simulink model "Project"  (R2020a)
settings: Solver=FixedStepDiscrete  StartTime=0.0  StopTime=10.0  FixedStep=1.0  RelTol=1e-3
libraries: simulink x4
settings Model: Creator=Sajad  LastModifiedBy=alireza
settings OptimizationCC: DefaultParameterBehavior=Inlined  UseDivisionForNetSlopeComputation=on  GainParamInheritBuiltInType=on  UseFloatMulNetSlope=on  InlineInvariantSignals=on  PassReuseOutputArgsAs=Individual arguments  ZeroExternalMemoryAtStartup=off  ZeroInternalMemoryAtStartup=off  NoFixptDivByZeroProtection=on  EfficientFloat2IntCast=on  LifeSpan=1  OptimizeBlockOrder=speed  DifferentSizesBufferReuse=on  EfficientTunableParamExpr=on
settings DebuggingCC: ParameterTunabilityLossMsg=error
settings HardwareCC: ProdBitPerInt=16  ProdBitPerPointer=16  ProdBitPerSizeT=16  ProdBitPerPtrDiffT=16  ProdLargestAtomicFloat=None  ProdWordSize=8  ProdLongLongMode=on  ProdHWDeviceType=Atmel->AVR
settings SFSimCC: MATLABDynamicMemAlloc=off  CustomCodeUndefinedFunction=UseInterfaceOnly
settings RTWCC: SystemTargetFile=ert.tlc  GenCodeOnly=on  TemplateMakefile=ert_default_tmf  GenerateReport=on  IncludeHyperlinkInReport=on  LaunchReport=on  TargetLang=C++  GenerateTraceInfo=on  GenerateTraceReport=on  GenerateTraceReportSl=on  GenerateTraceReportSf=on  GenerateTraceReportEml=on
settings CodeAppCC: ForceParamTrailComments=on  IgnoreCustomStorageClasses=off  OperatorAnnotations=on  SimulinkDataObjDesc=on  SFDataObjDesc=on  CustomSymbolStrGlobalVar=rt$N$M  CustomSymbolStrType=$N$M  CustomSymbolStrFcn=$N$M$F  CustomSymbolStrMacro=$N$M  InsertBlockDesc=on
settings ERTTargetCC: TargetLangStandard=C++03 (ISO)  GenerateSampleERTMain=on  IncludeMdlTerminateFcn=off  CombineSignalStateStructs=on  SupportAbsoluteTime=off  MultiInstanceERTCode=on  CodeInterfacePackaging=C++ class  PurelyIntegerCode=on  SupportComplex=off  SupportNonInlinedSFcns=on  InlinedParameterPlacement=NonHierarchical  RootIOFormat=Structure reference  ERTCustomFileTemplate=example_file_process.tlc  ERTFilePackagingFormat=CompactWithDataFile

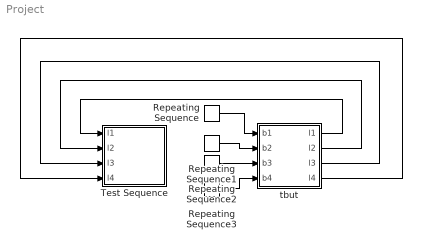
== system Project ==
  Repeating Sequence : simulink/Sources/Repeating Sequence  rep_seq_t=[0 1 2 3 4 5 6]  rep_seq_y=[0 1 1 0 0 0 0]
  Repeating Sequence1 : simulink/Sources/Repeating Sequence  rep_seq_t=[0 1 2 3 4 5 6]  rep_seq_y=[0 1 0 1 0 0 0]
  Repeating Sequence2 : simulink/Sources/Repeating Sequence  rep_seq_t=[0 1 2 3 4 5 6]  rep_seq_y=[0 1 0 0 1 0 0]
  Repeating Sequence3 : simulink/Sources/Repeating Sequence  rep_seq_t=[0 1 2 3 4 5 6]  rep_seq_y=[0 1 0 0 0 1 0]
  Test Sequence : Test Sequence  TreatAsAtomicUnit=on
  tbut : Stateflow chart  TreatAsAtomicUnit=on
  wires:
  tbut/1(l1) -> Test Sequence/1(l1)
  tbut/2(l2) -> Test Sequence/2(l2)
  tbut/3(l3) -> Test Sequence/3(l3)
  tbut/4(l4) -> Test Sequence/4(l4)
  Repeating Sequence/1 -> tbut/1(b1)
  Repeating Sequence3/1 -> tbut/4(b4)
  Repeating Sequence2/1 -> tbut/3(b3)
  Repeating Sequence1/1 -> tbut/2(b2)

== stateflow chart Project/tbut ==
  state fled_1 [parallel]
    settings: executionOrder=1
    state I
    state II
      l1 = ~l1;
    (default) -> fled_1.I
    fled_1.II -> fled_1.I [order 2]
    fled_1.I -> fled_1.II : [b1==1]
    fled_1.II -> fled_1.II [order 1] : [b1==1]
  state fled_2 [parallel]
    settings: executionOrder=2
    state I
    state II
      l2 = ~l2;
    (default) -> fled_2.I
    fled_2.II -> fled_2.I [order 2]
    fled_2.I -> fled_2.II : [b2==1]
    fled_2.II -> fled_2.II [order 1] : [b2==1]
  state fled_3 [parallel]
    settings: executionOrder=3
    state I
    state II
      l3 = ~l3;
    (default) -> fled_3.I
    fled_3.II -> fled_3.I [order 2]
    fled_3.I -> fled_3.II : [b3==1]
    fled_3.II -> fled_3.II [order 1] : [b3==1]
  state fled_4 [parallel]
    settings: executionOrder=4
    state I
    state II
      l4 = ~l4;
    (default) -> fled_4.I
    fled_4.II -> fled_4.I [order 2]
    fled_4.I -> fled_4.II : [b4==1]
    fled_4.II -> fled_4.II [order 1] : [b4==1]
  data: l1 output =false; l2 output =false; l3 output =false; l4 output =false; b1 input; b2 input; b3 input; b4 input

== stateflow chart Project/Test Sequence ==
  settings: stateMachineType=SIMPLIFIED_MACHINE
  state step_1
    verify(l1==false&& l2==false && l3==false && l4==false)
  state step_2
    verify(l1==true&& l2==true && l3==true && l4==true)
  state step_3
    verify(l1==false&& l2==true&& l3==true&& l4==true)
  state step_4
    verify(l1==false && l2==false && l3==true&& l4==true)
  state step_5
    verify(l1==false && l2==false&& l3==false&& l4==true)
  state step_6
    verify(l1==false&& l2==false && l3==false && l4==false)
  state step_7
  (default) -> step_1
  step_1 -> step_2 : [
      | after(1,sec)
      | ]
  step_2 -> step_3 : [
      | after(1,sec)
      | ]
  step_3 -> step_4 : [
      | after(1,sec)
      | ]
  step_4 -> step_5 : [
      | after(1,sec)
      | ]
  step_5 -> step_6 : [
      | after(1,sec)
      | ]
  step_6 -> step_7 : [
      | after(1,sec)
      | ]
  data: l1 input; l2 input; l3 input; l4 input
